simulink model "max_filter_test"  (R2021a)
settings: Solver=FixedStepDiscrete  StartTime=0.0  StopTime=60  FixedStep=0.1  RelTol=1e-3
libraries: pingcap x4
settings Model: Creator=tongjian  LastModifiedBy=tongjian

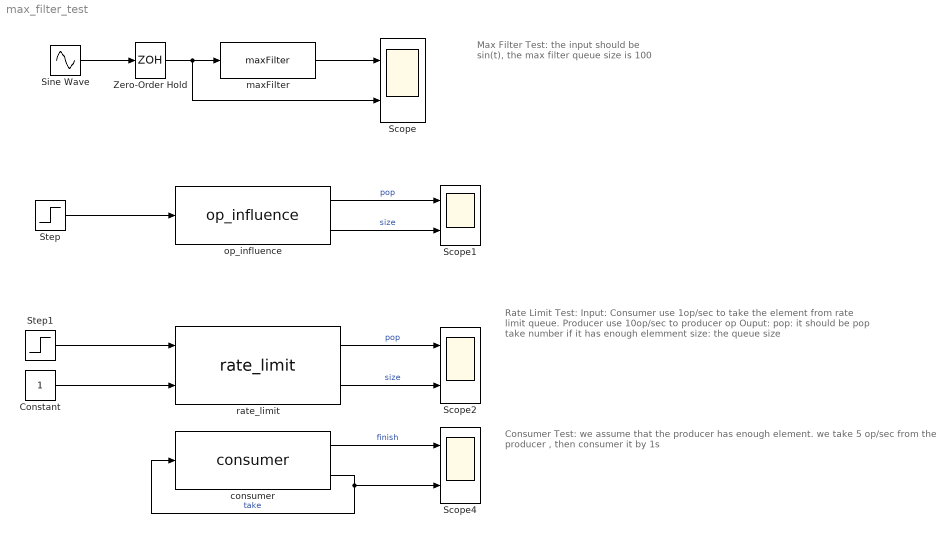
== system max_filter_test ==
  note: Consumer Test:
      |
      | we assume that the producer has enough element. we take 5 op/sec from the producer ,
      | then consumer it by 1s
  note: Rate Limit Test:
      |
      | Input:
      | 	Consumer use 1op/sec to take the element from rate limit queue.
      | 	Producer use 10op/sec to producer op
      |
      | Ouput:
      | 	pop: it should be pop take number if it has  enough elemment
      | 	size: the queue size
  note: Max Filter Test:
      | the input should be sin(t), the max filter queue size is 100
  Constant : Constant
  Scope{,1..2,4} (4 alike) : Scope  NumInputPorts=2
  Sine Wave : Sin  SampleTime=0
  Step : Step  Time=5  SampleTime=0
  Step1 : Step  Time=0  After=10  SampleTime=0
  Zero-Order Hold : ZeroOrderHold  SampleTime=-1
  consumer : pingcap/consumer  g_consumer_size=5  g_consumer_duration=1
  maxFilter : pingcap/maxFilter  g_n=100  g_Ts=1
  op_influence : pingcap/op_influence  g_store_limit=10  g_expired_time=500
  rate_limit : pingcap/rate_limit  g_store_limit=20
  wires:
  Sine Wave/1 -> Zero-Order Hold/1
  Zero-Order Hold/1 -> maxFilter/1, Scope/2
  maxFilter/1 -> Scope/1
  op_influence/1 -> Scope1/1  "pop"
  op_influence/2 -> Scope1/2  "size"
  Step/1 -> op_influence/1
  Step1/1 -> rate_limit/1
  Constant/1 -> rate_limit/2
  rate_limit/2 -> Scope2/2  "size"
  rate_limit/1 -> Scope2/1  "pop"
  consumer/2 -> Scope4/2, consumer/1  "take"
  consumer/1 -> Scope4/1  "finish"
